simulink model "UUV_Dyn_simulink"  (R2022a)
settings: Solver=VariableStepAuto  StartTime=0.0  StopTime=50.0  RelTol=1e-3
values from neighbouring files (symbols this model uses):
  eta_0 = [0; 0; 0; 0; 0; 0]    [UUV_Dyn_simulink_Animation.m]
  M_inv = inv(M)    [UUV_Dyn_simulink_Animation.m]
  V0 = [0; 0; 0; 0; 0; 0]    [UUV_Dyn_simulink_Animation.m]
settings Model: Creator=Sushmanth Sai G  LastModifiedBy=G_Sushmanth_Sai
settings DebuggingCC: UnconnectedInputMsg=warning  UnconnectedOutputMsg=warning  UnconnectedLineMsg=warning
settings RTWCC: DLArmComputeVersion=19.05

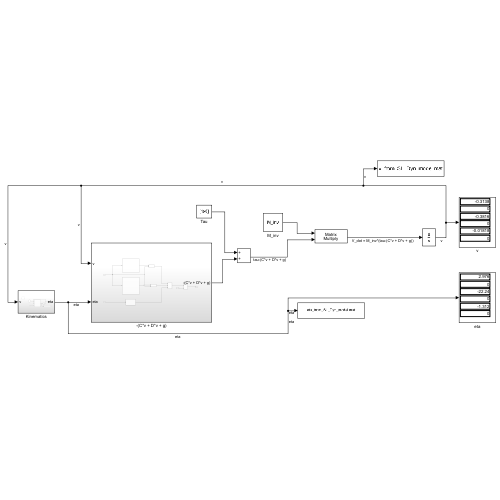
[thumbnail: Simulink's stored preview of the top-level diagram]
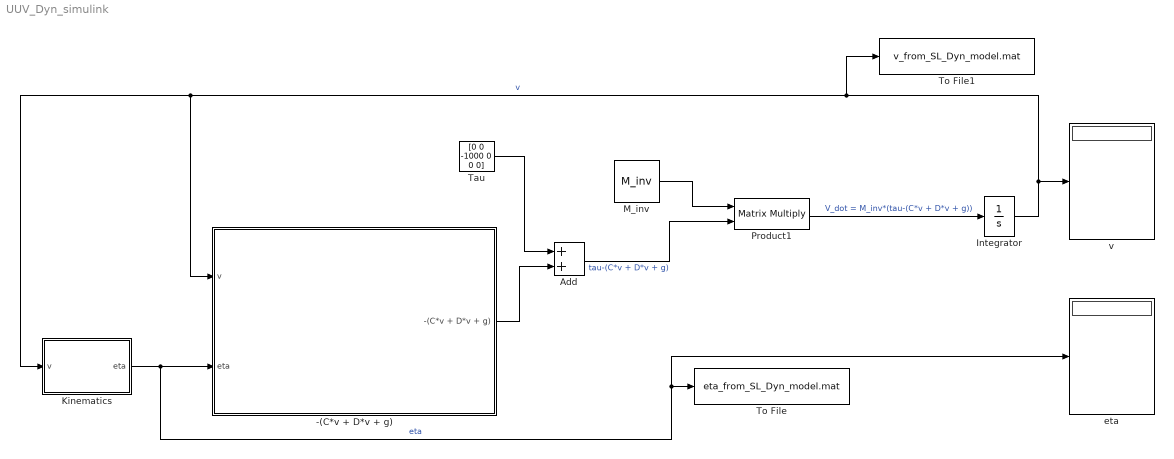
== system UUV_Dyn_simulink ==
  -(C*v + D*v + g) : Subsystem
  Add : Sum
  Integrator : Integrator  InitialCondition=V0
  Kinematics : Subsystem
  M_inv : Constant  Value=M_inv
  Product1 : Product  Multiplication=Matrix(*)
  Tau : Constant  Value=[0 0 -1000 0 0 0]
  To File : ToFile  Filename=eta_from_SL_Dyn_model.mat  MatrixName=eta
  To File1 : ToFile  Filename=v_from_SL_Dyn_model.mat  MatrixName=v
  eta : Display
  v : Display
  wires:
  -(C*v + D*v + g)/1(-(C*v + D*v + g)) -> Add/2
  Add/1 -> Product1/2  "tau-(C*v + D*v + g)"
  M_inv/1 -> Product1/1
  Product1/1 -> Integrator/1  "V_dot = M_inv*(tau-(C*v + D*v + g))"
  Kinematics/1(eta) -> To File/1, eta/1, -(C*v + D*v + g)/2(eta)  "eta"
  Integrator/1 -> To File1/1, Kinematics/1(v), -(C*v + D*v + g)/1(v), v/1  "v"
  Tau/1 -> Add/1

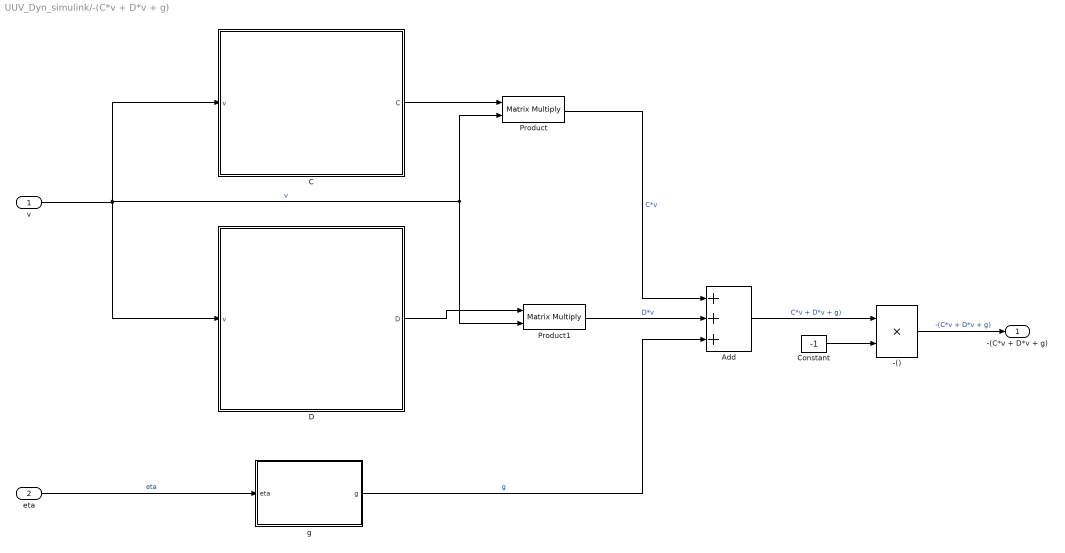
== system UUV_Dyn_simulink/-(C*v + D*v + g) ==
  v : Inport
  eta : Inport  Port=2
  -() : Product  Inputs=**
  Add : Sum  Inputs=+++
  C : Subsystem
  Constant : Constant  Value=-1
  D : Subsystem
  Product : Product  Multiplication=Matrix(*)
  Product1 : Product  Multiplication=Matrix(*)
  g : Subsystem
  -(C*v + D*v + g) : Outport
  wires:
  g/1(g) -> Add/3  "g"
  Constant/1 -> -()/2
  D/1(D) -> Product1/1
  C/1(C) -> Product/1
  Product/1 -> Add/1  "C*v"
  Add/1 -> -()/1  "C*v + D*v + g)"
  -()/1 -> -(C*v + D*v + g)/1  "-(C*v + D*v + g)"
  eta/1 -> g/1(eta)  "eta"
  v/1 -> Product1/2, Product/2, C/1(v), D/1(v)  "v"
  Product1/1 -> Add/2  "D*v"

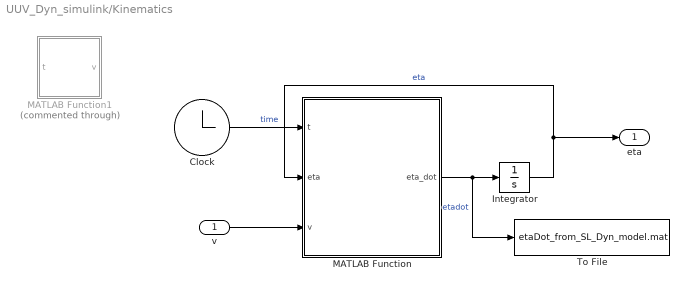
== system UUV_Dyn_simulink/Kinematics ==
  v : Inport
  Clock : Clock
  Integrator : Integrator  InitialCondition=eta_0
  MATLAB Function : MATLAB Function  TreatAsAtomicUnit=on
  MATLAB Function1 : MATLAB Function  Commented=through  TreatAsAtomicUnit=on
  To File : ToFile  Filename=etaDot_from_SL_Dyn_model.mat  MatrixName=etaDot
  eta : Outport
  wires:
  Clock/1 -> MATLAB Function/1(t)  "time"
  MATLAB Function/1(eta_dot) -> To File/1, Integrator/1  "etadot"
  Integrator/1 -> eta/1, MATLAB Function/2(eta)  "eta"
  v/1 -> MATLAB Function/3(v)

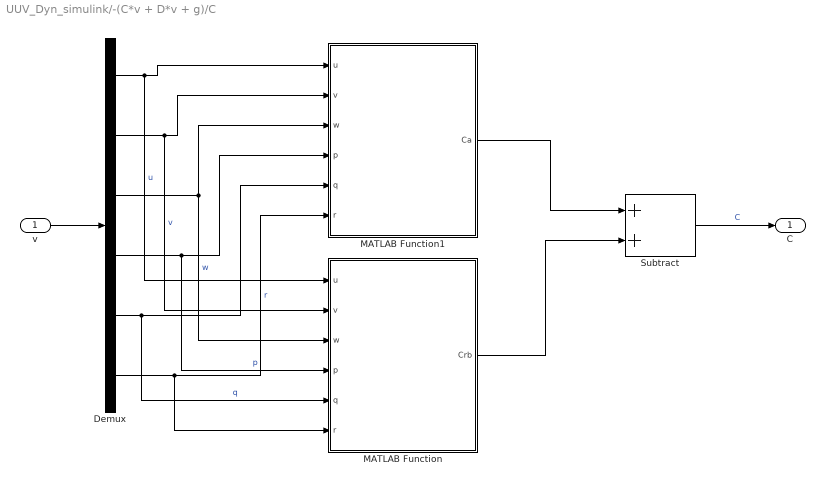
== system UUV_Dyn_simulink/-(C*v + D*v + g)/C ==
  v : Inport
  Demux : Demux  Outputs=6
  MATLAB Function : MATLAB Function  TreatAsAtomicUnit=on
  MATLAB Function1 : MATLAB Function  TreatAsAtomicUnit=on
  Subtract : Sum
  C : Outport
  wires:
  Demux/5 -> MATLAB Function/5(q), MATLAB Function1/5(q)  "q"
  Demux/6 -> MATLAB Function/6(r), MATLAB Function1/6(r)  "r"
  MATLAB Function/1(Crb) -> Subtract/2
  Demux/3 -> MATLAB Function/3(w), MATLAB Function1/3(w)  "w"
  Subtract/1 -> C/1  "C"
  Demux/1 -> MATLAB Function/1(u), MATLAB Function1/1(u)  "u"
  Demux/2 -> MATLAB Function/2(v), MATLAB Function1/2(v)  "v"
  Demux/4 -> MATLAB Function/4(p), MATLAB Function1/4(p)  "p"
  MATLAB Function1/1(Ca) -> Subtract/1
  v/1 -> Demux/1

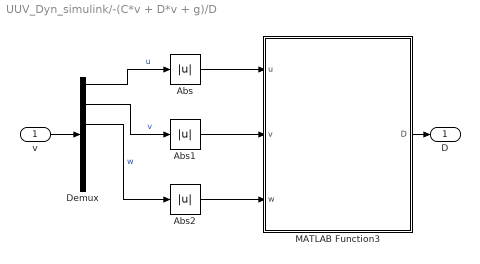
== system UUV_Dyn_simulink/-(C*v + D*v + g)/D ==
  v : Inport
  Abs : Abs  SaturateOnIntegerOverflow=off
  Abs1 : Abs  SaturateOnIntegerOverflow=off
  Abs2 : Abs  SaturateOnIntegerOverflow=off
  Demux : Demux  Outputs=6
  MATLAB Function3 : MATLAB Function  TreatAsAtomicUnit=on
  D : Outport
  wires:
  Demux/3 -> Abs2/1  "w"
  Demux/1 -> Abs/1  "u"
  Abs/1 -> MATLAB Function3/1(u)
  Abs2/1 -> MATLAB Function3/3(w)
  Abs1/1 -> MATLAB Function3/2(v)
  MATLAB Function3/1(D) -> D/1
  Demux/2 -> Abs1/1  "v"
  v/1 -> Demux/1

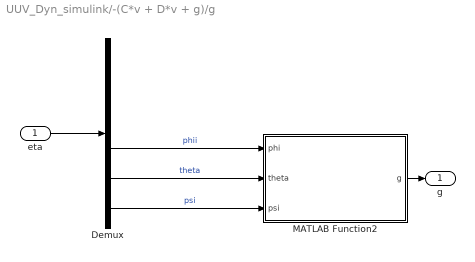
== system UUV_Dyn_simulink/-(C*v + D*v + g)/g ==
  eta : Inport
  Demux : Demux  Outputs=6
  MATLAB Function2 : MATLAB Function  TreatAsAtomicUnit=on
  g : Outport
  wires:
  Demux/6 -> MATLAB Function2/3(psi)  "psi"
  Demux/5 -> MATLAB Function2/2(theta)  "theta"
  Demux/4 -> MATLAB Function2/1(phi)  "phii"
  eta/1 -> Demux/1
  MATLAB Function2/1(g) -> g/1

== matlab function UUV_Dyn_simulink/Kinematics/MATLAB Function1 ==
  data: t input; v output
function v = f_v(t)
v = [0.5
     0
     0
     2*pi/10
     0
     0];
end

== matlab function UUV_Dyn_simulink/Kinematics/MATLAB Function ==
  data: t input; eta_dot output; eta input; v input
function eta_dot = V_P (t,eta,v)

phi = eta(4);
theta = eta(5);
psi = eta(6);

eta_dot = zeros(6,1);

Cpsi = [cos(psi) -sin(psi) 0
        sin(psi)  cos(psi) 0
        0          0       1];

Ctheta = [cos(theta)   0   sin(theta)
           0           1      0   
         -sin(theta)   0   cos(theta)];

Cphi = [1    0         0
        0 cos(phi) -sin(phi)
        0 sin(phi) cos(phi)];

J1 = Cpsi*Ctheta*Cphi;

J2= [1  sin(phi)*tan(theta)  cos(phi)*tan(theta)
     0      cos(phi)              -sin(phi)
     0 sin(phi)/cos(theta)   cos(phi)/cos(theta)]; 

J = [J1 zeros(3,3)
    zeros(3,3) J2];

eta_dot = J*v;

end

== matlab function UUV_Dyn_simulink/-(C*v + D*v + g)/C/MATLAB Function ==
  data: u input; Crb output; v input; w input; p input; q input; r input
function Crb = Mat_gen(u,v,w,p,q,r)


Crb = [     0                  0           0            0           32.16*q + 1462*w       32.16*r - 1462*v
            0                  0           0         -1462*w          -32.16*p                  1462*u
            0                  0           0          1462*v           -1462*u                 -32.16*p
            0                1462*w      -1462*v         0             2848.97*r              -1850.34*q
        -32.16*q - 1462*w    32.16*p     1462*u      -2848.97*r            0                   498.63*p
        -32.16*r + 1462*v    -1462*u     32.16*p      1850.34*q       -498.63*p                   0        ];

== matlab function UUV_Dyn_simulink/-(C*v + D*v + g)/C/MATLAB Function1 ==
  data: u input; Ca output; v input; w input; p input; q input; r input

function Ca= Mat_gen(u,v,w,p,q,r)


Ca = [            0                        0                              0                        0            7040.36*w - 277.20*q      -1049.21*v + 996.04*r
                  0                        0                              0             -7040.36*w + 277.20*q             0                       323.10*u
                  0                        0                              0              1049.21*v - 996.04*r         -323.10*u                      0
                  0              7040.36*w - 277.20*q          -1049.21*v + 996.04*r               0            -996.04*v + 8584.25*r      -277.20*w + 7045.28*q
       -7040.36*w + 277.20*q               0                           323.10*u          996.04*v - 8584.25*r             0                       645.85*p
        1049.21*v - 996.04*r           -323.10*u                          0             -277.20*w + 7045.28*q        -645.85*p                       0            ];

== matlab function UUV_Dyn_simulink/-(C*v + D*v + g)/g/MATLAB Function2 ==
  data: phi input; theta input; g output; psi input
function g = fcn(phi,theta,psi)

g = [           -49*sin(theta)
            49*cos(theta)*sin(phi)
            49*cos(theta)*cos(phi)
          215.87*cos(theta)*sin(phi)
    215.87*sin(theta) - 1.1*cos(theta)*cos(phi)
           1.1*cos(theta)*sin(phi)              ];

== matlab function UUV_Dyn_simulink/-(C*v + D*v + g)/D/MATLAB Function3 ==
  data: u input; D output; v input; w input
function D = Mat_gen(u,v,w)


D =   [ 0.25*ro*pi*rad^2*cdx*u^2                  0                                 0

                  0                    0.5*ro*2*rad*len*cdy*v^2                     0

                  0                               0                                 0 ];
